simulink model "do178b_dhc2"  (R2012b)
settings: Solver=ode23  StartTime=0.0  StopTime=25  MaxStep=1/40  RelTol=1e-2  AbsTol=1e-3
PreLoadFcn:
  | load asbdhc2_init;
  | Autopilot_bus;
undefined symbols (not defined in the file or in its folder): beaver_b, beaver_c, beaver_init_p, beaver_init_pitch, beaver_init_q, beaver_init_r, beaver_init_roll, beaver_mass, Cl0, Cl_alpha2_dpt, Cl_beta, Cl_da, Cl_da_alpha, Cl_dr, Cl_p, Cl_r, Cm0, Cm_alpha, Cm_alpha2, Cm_beta2, Cm_de, Cm_df, Cm_dpt, Cm_q, Cm_r, Cn0, Cn_beta, Cn_beta3, Cn_da, Cn_dpt3, Cn_dr, Cn_p, Cn_q, Cn_r, Cx0, Cx_alpha, Cx_alpha2, Cx_alpha3, Cx_df, Cx_df_alpha, Cx_dpt, Cx_dpt2_alpha, Cx_dr, Cx_q, Cy0, Cy_beta, Cy_da, Cy_dr, Cy_dr_alpha, Cy_p, Cy_r, Cz0, Cz_alpha, Cz_alpha3, Cz_de, Cz_de_beta, Cz_df, Cz_df_alpha, Cz_dpt, Cz_q ... (+9)
libraries: aerolibconvert2 x6, simulink x6, aerolibobsolete x4, aerolibasang x3, aerolibwind2 x3, aerolib6dof2 x1, aerolibadyn x1, aerolibatmos2 x1
(part 2 of 2)

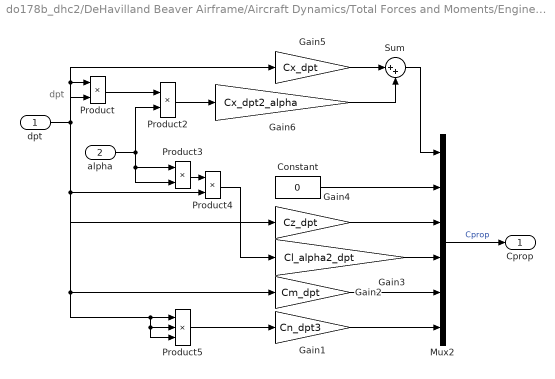
== system do178b_dhc2/DeHavilland Beaver Airframe/Aircraft Dynamics/Total Forces and Moments/Engine /eng ==
  note: dpt
  dpt : Inport
  alpha : Inport  Port=2
  Constant : Constant  Value=0
  Gain1 : Gain  Gain=Cn_dpt3  SaturateOnIntegerOverflow=on  OutDataTypeStr=Inherit: Same as input  ParamDataTypeStr=Inherit: Same as input
  Gain2 : Gain  Gain=Cm_dpt  SaturateOnIntegerOverflow=on  OutDataTypeStr=Inherit: Same as input  ParamDataTypeStr=Inherit: Same as input
  Gain3 : Gain  Gain=Cl_alpha2_dpt  SaturateOnIntegerOverflow=on  OutDataTypeStr=Inherit: Same as input  ParamDataTypeStr=Inherit: Same as input
  Gain4 : Gain  Gain=Cz_dpt  SaturateOnIntegerOverflow=on  OutDataTypeStr=Inherit: Same as input  ParamDataTypeStr=Inherit: Same as input
  Gain5 : Gain  Gain=Cx_dpt  SaturateOnIntegerOverflow=on  OutDataTypeStr=Inherit: Same as input  ParamDataTypeStr=Inherit: Same as input
  Gain6 : Gain  Gain=Cx_dpt2_alpha  SaturateOnIntegerOverflow=on  OutDataTypeStr=Inherit: Same as input  ParamDataTypeStr=Inherit: Same as input
  Mux2 : Mux  Inputs=6
  Product{,2..4} (4 alike) : Product  SaturateOnIntegerOverflow=on  OutDataTypeStr=Inherit: Same as first input
  Product5 : Product  Inputs=3  SaturateOnIntegerOverflow=on  OutDataTypeStr=Inherit: Same as first input
  Sum : Sum  Inputs=|++  SaturateOnIntegerOverflow=on
  Cprop : Outport
  wires:
  Product5/1 -> Gain1/1
  Sum/1 -> Mux2/1
  Gain6/1 -> Sum/2
  Gain5/1 -> Sum/1
  Constant/1 -> Mux2/2
  Gain4/1 -> Mux2/3
  Gain3/1 -> Mux2/4
  Gain2/1 -> Mux2/5
  Gain1/1 -> Mux2/6
  Product4/1 -> Gain3/1
  Product2/1 -> Gain6/1
  dpt/1 -> Gain5/1, Product5/3, Product5/2, Product5/1, Gain2/1, Gain4/1, Product/2, Product/1, Product4/2
  alpha/1 -> Product2/2, Product3/1, Product3/2
  Mux2/1 -> Cprop/1  "Cprop"
  Product/1 -> Product2/1
  Product3/1 -> Product4/1

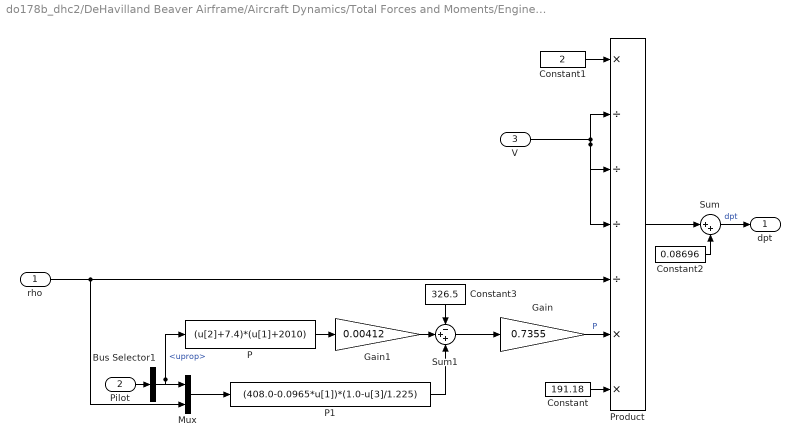
== system do178b_dhc2/DeHavilland Beaver Airframe/Aircraft Dynamics/Total Forces and Moments/Engine /pow ==
  rho : Inport
  Pilot : Inport  Port=2
  V : Inport  Port=3
  Bus Selector1 : BusSelector  OutputSignals=uprop
  Constant : Constant  Value=191.18
  Constant1 : Constant  Value=2
  Constant2 : Constant  Value=0.08696
  Constant3 : Constant  Value=326.5
  Gain : Gain  Gain=0.7355  SaturateOnIntegerOverflow=on  OutDataTypeStr=Inherit: Same as input  ParamDataTypeStr=Inherit: Same as input
  Gain1 : Gain  Gain=0.00412  SaturateOnIntegerOverflow=on  OutDataTypeStr=Inherit: Same as input  ParamDataTypeStr=Inherit: Same as input
  Mux : Mux  Inputs=2
  P : Fcn  Expr=(u[2]+7.4)*(u[1]+2010)
  P1 : Fcn  Expr=(408.0-0.0965*u[1])*(1.0-u[3]/1.225)
  Product : Product  Inputs=*////**  SaturateOnIntegerOverflow=on  OutDataTypeStr=Inherit: Same as first input
  Sum : Sum  Inputs=|++  SaturateOnIntegerOverflow=on
  Sum1 : Sum  Inputs=-++  SaturateOnIntegerOverflow=on
  dpt : Outport
  wires:
  P1/1 -> Sum1/3
  Constant3/1 -> Sum1/1
  Gain1/1 -> Sum1/2
  Mux/1 -> P1/1
  Sum1/1 -> Gain/1
  P/1 -> Gain1/1
  Gain/1 -> Product/6  "P"
  rho/1 -> Mux/2, Product/5
  Sum/1 -> dpt/1  "dpt"
  V/1 -> Product/4, Product/3, Product/2
  Bus Selector1/1 -> Mux/1, P/1  "<uprop>"
  Constant/1 -> Product/7
  Constant1/1 -> Product/1
  Product/1 -> Sum/1
  Constant2/1 -> Sum/2
  Pilot/1 -> Bus Selector1/1

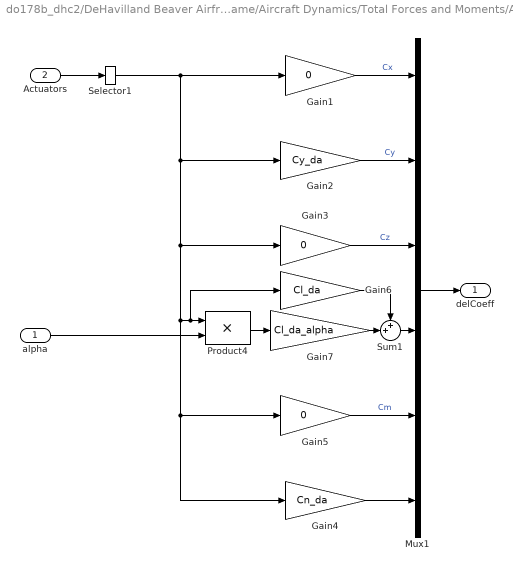
== system do178b_dhc2/DeHavilland Beaver Airframe/Aircraft Dynamics/Total Forces and Moments/Aerodynamics/Actuator Increments/Aileron ==
  alpha : Inport
  Actuators : Inport  Port=2
  Gain1 : Gain  Gain=0  SaturateOnIntegerOverflow=on  OutDataTypeStr=Inherit: Same as input  ParamDataTypeStr=Inherit: Same as input
  Gain2 : Gain  Gain=Cy_da  SaturateOnIntegerOverflow=on  OutDataTypeStr=Inherit: Same as input  ParamDataTypeStr=Inherit: Same as input
  Gain3 : Gain  Gain=0  SaturateOnIntegerOverflow=on  OutDataTypeStr=Inherit: Same as input  ParamDataTypeStr=Inherit: Same as input
  Gain4 : Gain  Gain=Cn_da  SaturateOnIntegerOverflow=on  OutDataTypeStr=Inherit: Same as input  ParamDataTypeStr=Inherit: Same as input
  Gain5 : Gain  Gain=0  SaturateOnIntegerOverflow=on  OutDataTypeStr=Inherit: Same as input  ParamDataTypeStr=Inherit: Same as input
  Gain6 : Gain  Gain=Cl_da  SaturateOnIntegerOverflow=on  OutDataTypeStr=Inherit: Same as input  ParamDataTypeStr=Inherit: Same as input
  Gain7 : Gain  Gain=Cl_da_alpha  SaturateOnIntegerOverflow=on  OutDataTypeStr=Inherit: Same as input  ParamDataTypeStr=Inherit: Same as input
  Mux1 : Mux  Inputs=6
  Product4 : Product  SaturateOnIntegerOverflow=on  InputSameDT=on  OutDataTypeStr=Inherit: Same as first input
  Selector1 : Selector  InputPortWidth=4  IndexOptions=Index vector (dialog)  Indices=2  OutputSizes=1
  Sum1 : Sum  Inputs=++|  SaturateOnIntegerOverflow=on
  delCoeff : Outport
  wires:
  Gain6/1 -> Sum1/1
  Sum1/1 -> Mux1/4
  Gain7/1 -> Sum1/2
  Product4/1 -> Gain7/1
  Gain1/1 -> Mux1/1  "Cx"
  alpha/1 -> Product4/2
  Actuators/1 -> Selector1/1
  Mux1/1 -> delCoeff/1
  Gain2/1 -> Mux1/2  "Cy"
  Gain3/1 -> Mux1/3  "Cz"
  Gain5/1 -> Mux1/5  "Cm"
  Gain4/1 -> Mux1/6
  Selector1/1 -> Gain1/1, Gain2/1, Gain3/1, Gain6/1, Product4/1, Gain5/1, Gain4/1

== system do178b_dhc2/DeHavilland Beaver Airframe/Aircraft Dynamics/Total Forces and Moments/Aerodynamics/Actuator Increments/Elevator ==
  Actuators : Inport
  Beta : Inport  Port=2
  Constant1 : Constant  Value=0
  Gain1 : Gain  Gain=Cz_de  SaturateOnIntegerOverflow=on  OutDataTypeStr=Inherit: Same as input  ParamDataTypeStr=Inherit: Same as input
  Gain2 : Gain  Gain=Cz_de_beta  SaturateOnIntegerOverflow=on  OutDataTypeStr=Inherit: Same as input  ParamDataTypeStr=Inherit: Same as input
  Gain3 : Gain  Gain=Cm_de  SaturateOnIntegerOverflow=on  OutDataTypeStr=Inherit: Same as input  ParamDataTypeStr=Inherit: Same as input
  Mux1 : Mux  Inputs=6
  Product4 : Product  Inputs=3  SaturateOnIntegerOverflow=on  InputSameDT=on  OutDataTypeStr=Inherit: Same as first input
  Selector1 : Selector  InputPortWidth=4  IndexOptions=Index vector (dialog)  Indices=1  OutputSizes=1
  Sum1 : Sum  SaturateOnIntegerOverflow=on
  delCoeff : Outport
  wires:
  Gain3/1 -> Mux1/5
  Gain1/1 -> Sum1/2
  Gain2/1 -> Sum1/1
  Sum1/1 -> Mux1/3
  Product4/1 -> Gain2/1
  Beta/1 -> Product4/2, Product4/1
  Mux1/1 -> delCoeff/1
  Selector1/1 -> Gain3/1, Gain1/1, Product4/3
  Constant1/1 -> Mux1/1, Mux1/2, Mux1/4, Mux1/6
  Actuators/1 -> Selector1/1

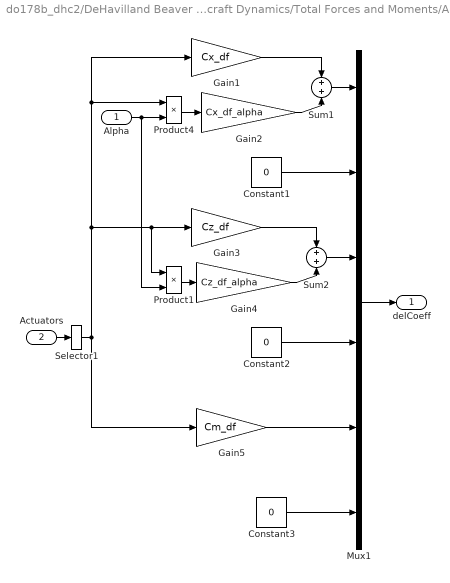
== system do178b_dhc2/DeHavilland Beaver Airframe/Aircraft Dynamics/Total Forces and Moments/Aerodynamics/Actuator Increments/Flap ==
  Alpha : Inport
  Actuators : Inport  Port=2
  Constant1 : Constant  Value=0
  Constant2 : Constant  Value=0
  Constant3 : Constant  Value=0
  Gain1 : Gain  Gain=Cx_df  SaturateOnIntegerOverflow=on  OutDataTypeStr=Inherit: Same as input  ParamDataTypeStr=Inherit: Same as input
  Gain2 : Gain  Gain=Cx_df_alpha  SaturateOnIntegerOverflow=on  OutDataTypeStr=Inherit: Same as input  ParamDataTypeStr=Inherit: Same as input
  Gain3 : Gain  Gain=Cz_df  SaturateOnIntegerOverflow=on  OutDataTypeStr=Inherit: Same as input  ParamDataTypeStr=Inherit: Same as input
  Gain4 : Gain  Gain=Cz_df_alpha  SaturateOnIntegerOverflow=on  OutDataTypeStr=Inherit: Same as input  ParamDataTypeStr=Inherit: Same as input
  Gain5 : Gain  Gain=Cm_df  SaturateOnIntegerOverflow=on  OutDataTypeStr=Inherit: Same as input  ParamDataTypeStr=Inherit: Same as input
  Mux1 : Mux  Inputs=6
  Product1 : Product  SaturateOnIntegerOverflow=on  InputSameDT=on  OutDataTypeStr=Inherit: Same as first input
  Product4 : Product  SaturateOnIntegerOverflow=on  InputSameDT=on  OutDataTypeStr=Inherit: Same as first input
  Selector1 : Selector  InputPortWidth=4  IndexOptions=Index vector (dialog)  Indices=4  OutputSizes=1
  Sum1 : Sum  SaturateOnIntegerOverflow=on
  Sum2 : Sum  SaturateOnIntegerOverflow=on
  delCoeff : Outport
  wires:
  Selector1/1 -> Gain1/1, Product4/1, Product1/1, Gain3/1, Gain5/1
  Actuators/1 -> Selector1/1
  Gain5/1 -> Mux1/5
  Gain3/1 -> Sum2/1
  Gain4/1 -> Sum2/2
  Product1/1 -> Gain4/1
  Gain1/1 -> Sum1/1
  Gain2/1 -> Sum1/2
  Product4/1 -> Gain2/1
  Alpha/1 -> Product1/2, Product4/2
  Mux1/1 -> delCoeff/1
  Sum1/1 -> Mux1/1
  Sum2/1 -> Mux1/3
  Constant1/1 -> Mux1/2
  Constant2/1 -> Mux1/4
  Constant3/1 -> Mux1/6

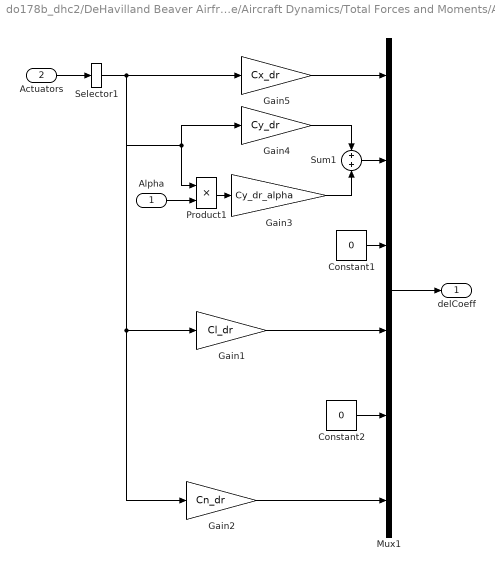
== system do178b_dhc2/DeHavilland Beaver Airframe/Aircraft Dynamics/Total Forces and Moments/Aerodynamics/Actuator Increments/Rudder ==
  Alpha : Inport
  Actuators : Inport  Port=2
  Constant1 : Constant  Value=0
  Constant2 : Constant  Value=0
  Gain1 : Gain  Gain=Cl_dr  SaturateOnIntegerOverflow=on  OutDataTypeStr=Inherit: Same as input  ParamDataTypeStr=Inherit: Same as input
  Gain2 : Gain  Gain=Cn_dr  SaturateOnIntegerOverflow=on  OutDataTypeStr=Inherit: Same as input  ParamDataTypeStr=Inherit: Same as input
  Gain3 : Gain  Gain=Cy_dr_alpha  SaturateOnIntegerOverflow=on  OutDataTypeStr=Inherit: Same as input  ParamDataTypeStr=Inherit: Same as input
  Gain4 : Gain  Gain=Cy_dr  SaturateOnIntegerOverflow=on  OutDataTypeStr=Inherit: Same as input  ParamDataTypeStr=Inherit: Same as input
  Gain5 : Gain  Gain=Cx_dr  SaturateOnIntegerOverflow=on  OutDataTypeStr=Inherit: Same as input  ParamDataTypeStr=Inherit: Same as input
  Mux1 : Mux  Inputs=6
  Product1 : Product  SaturateOnIntegerOverflow=on  InputSameDT=on  OutDataTypeStr=Inherit: Same as first input
  Selector1 : Selector  InputPortWidth=4  IndexOptions=Index vector (dialog)  Indices=3  OutputSizes=1
  Sum1 : Sum  SaturateOnIntegerOverflow=on
  delCoeff : Outport
  wires:
  Gain5/1 -> Mux1/1
  Gain4/1 -> Sum1/1
  Gain3/1 -> Sum1/2
  Gain1/1 -> Mux1/4
  Gain2/1 -> Mux1/6
  Product1/1 -> Gain3/1
  Alpha/1 -> Product1/2
  Mux1/1 -> delCoeff/1
  Actuators/1 -> Selector1/1
  Sum1/1 -> Mux1/2
  Constant1/1 -> Mux1/3
  Constant2/1 -> Mux1/5
  Selector1/1 -> Gain5/1, Gain4/1, Gain1/1, Gain2/1, Product1/1

== system do178b_dhc2/DeHavilland Beaver Airframe/Aircraft Dynamics/Total Forces and Moments/Aerodynamics/Body Rate Damping/p ==
  Constant1 : Constant  Value=0
  Constant2 : Constant  Value=Cy_p
  Constant3 : Constant  Value=Cl_p
  Constant4 : Constant  Value=Cn_p
  Mux1 : Mux  Inputs=6
  delCoeff : Outport
  wires:
  Constant2/1 -> Mux1/2
  Mux1/1 -> delCoeff/1
  Constant1/1 -> Mux1/5, Mux1/3, Mux1/1
  Constant4/1 -> Mux1/6
  Constant3/1 -> Mux1/4

== system do178b_dhc2/DeHavilland Beaver Airframe/Aircraft Dynamics/Total Forces and Moments/Aerodynamics/Body Rate Damping/q ==
  Constant1 : Constant  Value=0
  Constant2 : Constant  Value=Cz_q
  Constant3 : Constant  Value=Cx_q
  Constant4 : Constant  Value=Cm_q
  Constant5 : Constant  Value=Cn_q
  Mux1 : Mux  Inputs=6
  delCoeff : Outport
  wires:
  Constant2/1 -> Mux1/3
  Constant5/1 -> Mux1/6
  Constant1/1 -> Mux1/4, Mux1/2
  Constant4/1 -> Mux1/5
  Constant3/1 -> Mux1/1
  Mux1/1 -> delCoeff/1

== system do178b_dhc2/DeHavilland Beaver Airframe/Aircraft Dynamics/Total Forces and Moments/Aerodynamics/Body Rate Damping/r ==
  Constant : Constant  Value=0
  Constant1 : Constant  Value=Cy_r
  Constant2 : Constant  Value=Cl_r
  Constant3 : Constant  Value=Cm_r
  Constant4 : Constant  Value=Cn_r
  Mux1 : Mux  Inputs=6
  delCoeff : Outport
  wires:
  Constant3/1 -> Mux1/5
  Constant1/1 -> Mux1/2
  Constant4/1 -> Mux1/6
  Constant2/1 -> Mux1/4
  Constant/1 -> Mux1/3, Mux1/1
  Mux1/1 -> delCoeff/1
